simulink model "Day08"  (R2024b)
settings: Solver=VariableStepAuto  StartTime=0.0  StopTime=10.0  RelTol=1e-3
libraries: simulink x2
settings Model: Creator=jun_mac  LastModifiedBy=jun_mac

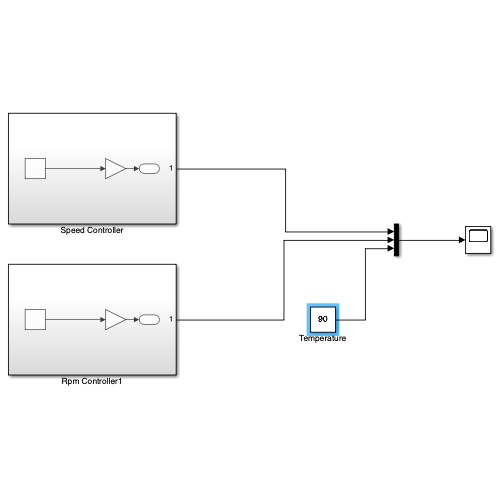
[thumbnail: Simulink's stored preview of the top-level diagram]
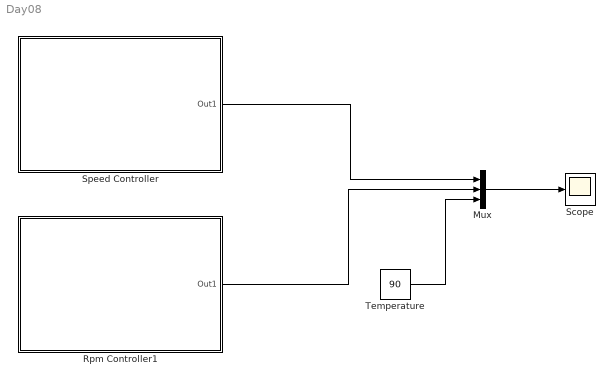
== system Day08 ==
  Mux : Mux  Inputs=3
  Rpm Controller1 : Subsystem
  Scope : Scope
  Speed Controller : Subsystem
  Temperature : Constant  Value=90
  wires:
  Mux/1 -> Scope/1
  Speed Controller/1(Out1) -> Mux/1
  Rpm Controller1/1(Out1) -> Mux/2
  Temperature/1 -> Mux/3

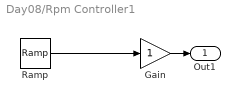
== system Day08/Rpm Controller1 ==
  Gain : Gain
  Ramp : simulink/Sources/Ramp  slope=100  start=0  InitialOutput=0
  Out1 : Outport
  wires:
  Gain/1 -> Out1/1
  Ramp/1 -> Gain/1

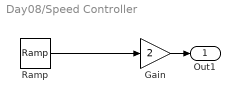
== system Day08/Speed Controller ==
  Gain : Gain  Gain=2
  Ramp : simulink/Sources/Ramp  slope=10  start=0  InitialOutput=0
  Out1 : Outport
  wires:
  Gain/1 -> Out1/1
  Ramp/1 -> Gain/1
